simulink model "wyp_most_3f"  (Simulink 9.3)
settings: Solver=FixedStepAuto  StartTime=0.0  StopTime=0.1  FixedStep=2e-4  MaxStep=2e-4  EnableMultiTasking=on
libraries: powerlib x18, powerlib_extras x5
settings Model: Creator=Teacher  LastModifiedBy=ogure
settings SolverCC: SolverResetMethod=Robust
settings DataIOCC: LimitDataPoints=on
settings OptimizationCC: InitFltsAndDblsToZero=on
settings DebuggingCC: SaveWithParameterizedLinksMsg=none  SignalResolutionControl=TryResolveAllWithWarning  SolverPrmCheckMsg=warning  MultiTaskDSMMsg=warning  MultiTaskCondExecSysMsg=none
settings GRTTargetCC: TargetFcnLib=ansi_tfl_tmw.mat  GeneratePreprocessorConditionals=Disable all
settings ConfigComp: CovSFcnEnable=off
settings SimscapeCC: SimscapeNormalizeSystem=off

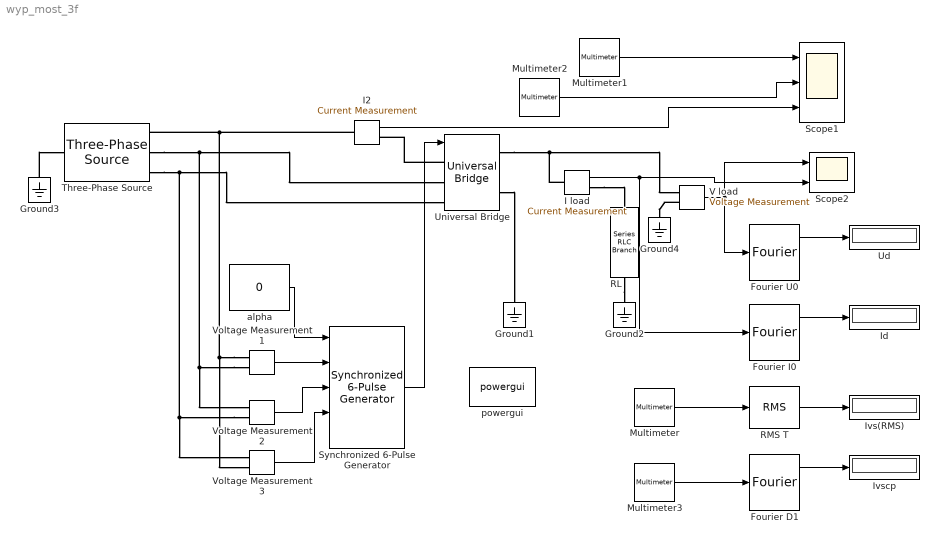
== system wyp_most_3f ==
  Fourier D1 : powerlib_extras/Measurements/Fourier  f1=50  n=0
      settings: SourceProductName=Simscape Electrical  SourceProductBaseCode=PS
  Fourier I0 : powerlib_extras/Measurements/Fourier  f1=300  n=0
      settings: SourceProductName=Simscape Electrical  SourceProductBaseCode=PS
  Fourier U0 : powerlib_extras/Measurements/Fourier  f1=300  n=0
      settings: SourceProductName=Simscape Electrical  SourceProductBaseCode=PS
  Ground{1..4} (4 alike) : powerlib/Elements/Ground  LConnTagsString=a
      settings: SourceProductName=Simscape Electrical
  I load : powerlib/Measurements/Current Measurement  PhasorSimulation=off  OutputType=Complex  PSBequivalent=0
      settings: SourceProductName=Simscape Electrical
  I2 : powerlib/Measurements/Current Measurement  PhasorSimulation=off  OutputType=Complex  PSBequivalent=0
      settings: SourceProductName=Simscape Electrical
  Id : Display
      settings: Decimation=3
  Ivs(RMS) : Display
      settings: Decimation=3
  Ivsср : Display
      settings: Decimation=3
  Multimeter : powerlib/Measurements/Multimeter  PhasorSimulation=off  OutputType=Complex  sel=11  L=16  Gain=1  yselected={'Isw1: Universal Bridge'};  PSBOutputType=1  PSBequivalent=0  AxesSetting=[0,0.1,-100,100]  Display=0  SavedBlockNames=-11
      settings: SourceProductName=Simscape Electrical
  Multimeter1 : powerlib/Measurements/Multimeter  PhasorSimulation=off  OutputType=Complex  sel=[1 4]  L=16  Gain=[1 1]  yselected={'Usw1: Universal Bridge','Usw4: Universal Bridge'};  PSBOutputType=1  PSBequivalent=0  AxesSetting=[0,0.1,-100,100]  Display=0  SavedBlockNames=-11
      settings: SourceProductName=Simscape Electrical
  Multimeter2 : powerlib/Measurements/Multimeter  PhasorSimulation=off  OutputType=Complex  sel=[11 14]  L=16  Gain=[1 1]  yselected={'Isw1: Universal Bridge','Isw4: Universal Bridge'};  PSBOutputType=1  PSBequivalent=0  AxesSetting=[0,0.1,-100,100]  Display=0  SavedBlockNames=-11
      settings: SourceProductName=Simscape Electrical
  Multimeter3 : powerlib/Measurements/Multimeter  PhasorSimulation=off  OutputType=Complex  sel=11  L=16  Gain=1  yselected={'Isw1: Universal Bridge'};  PSBOutputType=1  PSBequivalent=0  AxesSetting=[0,0.1,-100,100]  Display=0  SavedBlockNames=-11
      settings: SourceProductName=Simscape Electrical
  RL : powerlib/Elements/Series RLC Branch  LConnTagsString=__new0  RConnTagsString=__new0  BranchType=RL  Resistance=0.04  Inductance=530.5e-6  SetiL0=off  InitialCurrent=0  Capacitance=inf  Setx0=off  InitialVoltage=0  Measurements=None
      settings: SourceProductName=Simscape Electrical
  RMS T : powerlib_extras/Measurements/RMS  f1=50
      settings: SourceProductName=Simscape Electrical  SourceProductBaseCode=PS
  Scope1 : Scope  NumInputPorts=3
  Scope2 : Scope  NumInputPorts=2
  Synchronized 6-Pulse Generator : powerlib_extras/Control  Blocks/Synchronized 6-Pulse Generator  freq=50  pwidth=10  Double_Pulse=off
      settings: SourceProductName=Simscape Electrical  SourceProductBaseCode=PS
  Three-Phase Source : powerlib/Electrical Sources/Three-Phase Source  InternalConnection=Yn  VoltagePhases=off  Voltage=9.2*sqrt(3)  PhaseAngle=0  Voltage_phases=[25e3 25e3 25e3]/sqrt(3)  PhaseAngles_phases=[0 -120 +120]  Frequency=50  NonIdealSource=on  SpecifyImpedance=off  Resistance=0.69  Inductance=0  ShortCircuitLevel=100e6  BaseVoltage=9.2*sqrt(3)  XRratio=7  BusType=swing  Pref=0  Qref=0  Prefabc=[10e3, 10e3, 10e3]  Qrefabc=[0, 0, 0]  Qmin=-inf  Qmax=inf
      settings: SourceProductName=Simscape Electrical
  Ud : Display
      settings: Decimation=3
  Universal Bridge : powerlib/Power Electronics/Universal Bridge  Arms=3  SnubberResistance=1e6  SnubberCapacitance=1e-9  Device=Thyristors  Ron=1.05e-3  Lon=0  ForwardVoltages="[  0  0  ]"  ForwardVoltage=1.05  GTOparameters=[ 10e-6 , 20e-6 ]  IGBTparameters=[ 1e-6 , 2e-6 ]  Measurements=All voltages and currents  Measurements_2=None  converterType=Rectifier
      settings: SourceProductName=Simscape Electrical
  V load : powerlib/Measurements/Voltage Measurement  PhasorSimulation=off  OutputType=Complex  PSBequivalent=0
      settings: SourceProductName=Simscape Electrical
  Voltage Measurement1 : powerlib/Measurements/Voltage Measurement  PhasorSimulation=off  OutputType=Complex  PSBequivalent=0
      settings: SourceProductName=Simscape Electrical
  Voltage Measurement2 : powerlib/Measurements/Voltage Measurement  PhasorSimulation=off  OutputType=Complex  PSBequivalent=0
      settings: SourceProductName=Simscape Electrical
  Voltage Measurement3 : powerlib/Measurements/Voltage Measurement  PhasorSimulation=off  OutputType=Complex  PSBequivalent=0
      settings: SourceProductName=Simscape Electrical
  alpha : Constant  Value=0  VectorParams1D=off
  powergui : powerlib/powergui  Priority=1  SimulationMode=Discrete  SampleTime=2e-4  frequency=60  Iterations=50  frequencyindice=50  Pbase=100e6  ErrMax=1e-4  UnitsV=kV  UnitsW=MW  buscounter=0  FunctionMessages=off  echomessages=off  EnableUseOfTLC=off  CurrentSourceSwitches=on  DisableSnubberDevices=off  DisableRonSwitches=off  DisableVfSwitches=off  DisplayEquations=off  AutomaticDiscreteSolvers=off  SolverType=Tustin/Backward Euler (TBE)  Interpol=off  ExternalGateDelay=off  methode=off  Ts=100  x0status=blocks  SPID=off  SwTol=0  HookPort=off  NonlinearTolerance=0  nMaxIteration=15  ContinueOnMaxIteration=off  RestoreLinks=warning  ResistiveCurrentMeasurement=off  Frange=[0:2:500]  Ylog=off  Xlog=on  ShowGrid=off  save=off  variable=ZData  structure=0  ZoomFFT=off  StartTime=0.0  cycles=1  DisplayStyle=1  fundamental=60  FreqAxis=off  MaxFrequency=1000  frequencyindicesteady=1  RmsSteady=1  display=off
      settings: SourceProductName=Simscape Electrical
  wires:
  I load/1 -> Scope2/2, Fourier I0/1
  RMS T/1 -> Ivs(RMS)/1
  V load/1 -> Scope2/1, Fourier U0/1
  Multimeter/1 -> RMS T/1
  Multimeter2/1 -> Scope1/2
  Multimeter1/1 -> Scope1/1
  Multimeter3/1 -> Fourier D1/1
  Fourier D1/1 -> Ivsср/1
  Fourier I0/1 -> Id/1
  Fourier U0/1 -> Ud/1
  Synchronized 6-Pulse Generator/1 -> Universal Bridge/1
  alpha/1 -> Synchronized 6-Pulse Generator/1
  Voltage Measurement1/1 -> Synchronized 6-Pulse Generator/2
  Voltage Measurement3/1 -> Synchronized 6-Pulse Generator/4
  Voltage Measurement2/1 -> Synchronized 6-Pulse Generator/3
  I2/1 -> Scope1/3
  connections:
  Voltage Measurement1/LConn1 -- I2/LConn1 -- Three-Phase Source/RConn1 -- Voltage Measurement3/LConn2
  Universal Bridge/LConn1 -- I2/RConn1
  Voltage Measurement1/LConn2 -- Three-Phase Source/RConn2 -- Universal Bridge/LConn2 -- Voltage Measurement2/LConn1
  Voltage Measurement2/LConn2 -- Three-Phase Source/RConn3 -- Universal Bridge/LConn3 -- Voltage Measurement3/LConn1
  I load/LConn1 -- Universal Bridge/RConn1 -- V load/LConn1
  Universal Bridge/RConn2 -- Ground1/LConn1
  I load/RConn1 -- RL/LConn1
  RL/RConn1 -- Ground2/LConn1
  V load/LConn2 -- Ground4/LConn1
  Ground3/LConn1 -- Three-Phase Source/LConn1
